simulink model "model"  (R2020b)
settings: Solver=VariableStepAuto  StartTime=0.0  StopTime=10.0  RelTol=1e-3
model workspace (MAT data in the model file):
  C = Simulink.Parameter
  C.Value = 1e-05
  C.DataType = 'auto'
  C.Dimensions = [1 1]
  R = Simulink.Parameter
  R.Value = 10
  R.DataType = 'auto'
  R.Dimensions = [1 1]
settings Model: OrderedModelArguments=off  Creator=Lenovo  LastModifiedBy=Lenovo

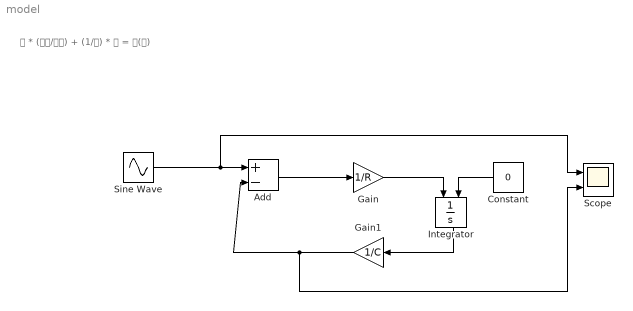
== system model ==
  note: 𝑅 * (𝑑𝑄/𝑑𝑡) + (1/𝐶) * 𝑄 = 𝐸(𝑡)
  Add : Sum  Inputs=+-
  Constant : Constant  Value=0
  Gain : Gain  Gain=1/R
  Gain1 : Gain  Gain=1/C
  Integrator : Integrator  InitialConditionSource=external
  Scope : Scope  NumInputPorts=2
  Sine Wave : Sin  SampleTime=0
  wires:
  Sine Wave/1 -> Scope/1, Add/1
  Add/1 -> Gain/1
  Integrator/1 -> Gain1/1
  Gain/1 -> Integrator/1
  Gain1/1 -> Scope/2, Add/2
  Constant/1 -> Integrator/2
